simulink model "Problem5"  (R2016a)
settings: Solver=VariableStepAuto  StartTime=0.0  StopTime=.2  RelTol=1e-3
values from neighbouring files (symbols this model uses):
  f_sw = 10e3    (= 10000)    [EE487_HW4.m]
  If_desired = Vbus/((P/2)*Maf*wr)    (= 1.9098593171)    [EE487_HW4.m]
  K_i_a = 100    [EE487_HW4.m]
  K_i_f = 100    [EE487_HW4.m]
  K_p_a = 100    [EE487_HW4.m]
  K_p_f = 100    [EE487_HW4.m]
  La = 1e-3    (= 0.001)    [EE487_HW4.m]
  Lf = 200e-3    (= 0.2)    [EE487_HW4.m]
  Maf = 40e-3    (= 0.04)    [EE487_HW4.m]
  P = 4    [EE487_HW4.m]
  Ra = 1e-3    (= 0.001)    [EE487_HW4.m]
  Rf = 20    [EE487_HW4.m]
  T_step = 5    [EE487_HW4.m]
  Vbus = 48    [EE487_HW4.m]
  wr = (2*pi*rpm)/60    (= 314.159265359)    [EE487_HW4.m]
libraries: dspsigops x3
settings Model: Creator=Seth Barger  LastModifiedBy=Seth Barger

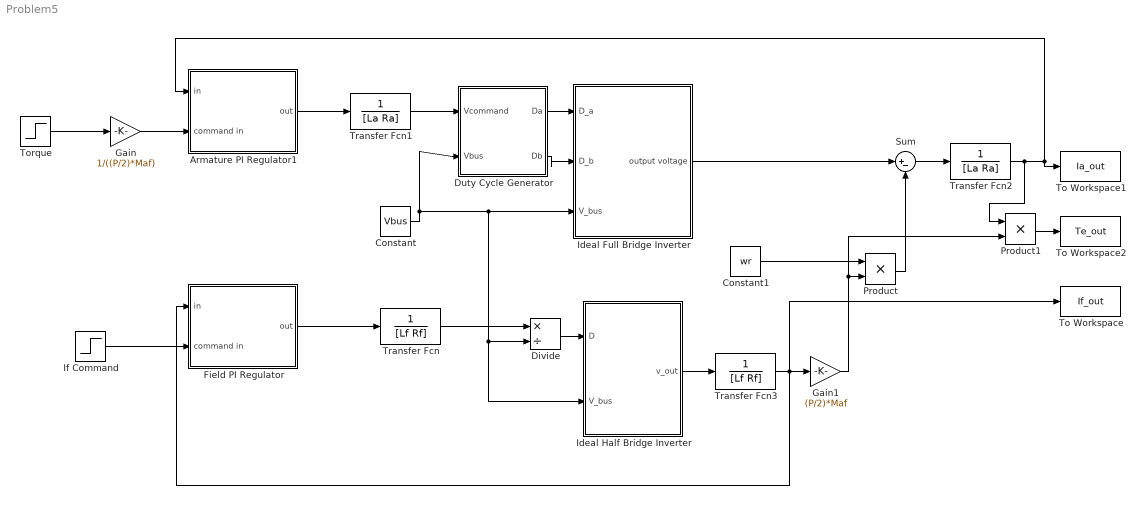
== system Problem5 ==
  Armature PI Regulator1 : Subsystem
  Constant : Constant  Value=Vbus
  Constant1 : Constant  Value=wr
  Divide : Product  Inputs=*/
  "Duty Cycle Generator " : Subsystem
  Field PI Regulator : Subsystem
  Gain : Gain  Gain=1/((P/2)*Maf)
  Gain1 : Gain  Gain=(P/2)*Maf
  "Ideal Half Bridge Inverter " : Subsystem
  "Ideal Full Bridge Inverter " : Subsystem
  If Command : Step  Time=.002  After=If_desired  SampleTime=0
  Product : Product
  Product1 : Product
  Sum : Sum  Inputs=|+-
  To Workspace : ToWorkspace  VariableName=If_out  SampleTime=-1
  To Workspace1 : ToWorkspace  VariableName=Ia_out  SampleTime=-1
  To Workspace2 : ToWorkspace  VariableName=Te_out  SampleTime=-1
  Torque : Step  Time=.002  After=T_step  SampleTime=0
  Transfer Fcn : TransferFcn  Denominator=[Lf Rf]
  Transfer Fcn1 : TransferFcn  Denominator=[La Ra]
  Transfer Fcn2 : TransferFcn  Denominator=[La Ra]
  Transfer Fcn3 : TransferFcn  Denominator=[Lf Rf]
  wires:
  "Duty Cycle Generator "/1(Da) -> "Ideal Full Bridge Inverter "/1(D_a)
  "Duty Cycle Generator "/2(Db) -> "Ideal Full Bridge Inverter "/2(D_b)
  Divide/1 -> "Ideal Half Bridge Inverter "/1(D)
  Constant/1 -> "Ideal Half Bridge Inverter "/2(V_bus), Divide/2, "Ideal Full Bridge Inverter "/3(V_bus), "Duty Cycle Generator "/2(Vbus)
  Field PI Regulator/1(out) -> Transfer Fcn/1
  Transfer Fcn/1 -> Divide/1
  Transfer Fcn1/1 -> "Duty Cycle Generator "/1(Vcommand)
  "Ideal Half Bridge Inverter "/1(v_out) -> Transfer Fcn3/1
  Transfer Fcn3/1 -> To Workspace/1, Gain1/1, Field PI Regulator/1(in)
  Transfer Fcn2/1 -> Product1/1, Armature PI Regulator1/1(in), To Workspace1/1
  If Command/1 -> Field PI Regulator/2(command in)
  Gain/1 -> Armature PI Regulator1/2(command in)
  Torque/1 -> Gain/1
  Armature PI Regulator1/1(out) -> Transfer Fcn1/1
  "Ideal Full Bridge Inverter "/1(output voltage) -> Sum/1
  Constant1/1 -> Product/1
  Product/1 -> Sum/2
  Sum/1 -> Transfer Fcn2/1
  Product1/1 -> To Workspace2/1
  Gain1/1 -> Product1/2, Product/2

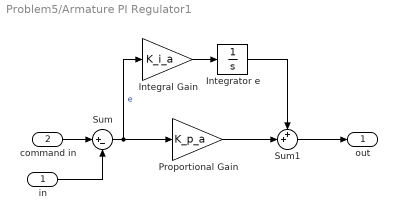
== system Problem5/Armature PI Regulator1 ==
  in : Inport
  command in : Inport  Port=2
  Integral Gain : Gain  Gain=K_i_a  SaturateOnIntegerOverflow=on  OutDataTypeStr=Inherit: Same as input  ParamDataTypeStr=Inherit: Same as input
  Integrator e : Integrator
  Proportional Gain : Gain  Gain=K_p_a  SaturateOnIntegerOverflow=on  OutDataTypeStr=Inherit: Same as input  ParamDataTypeStr=Inherit: Same as input
  Sum : Sum  Inputs=|+-  SaturateOnIntegerOverflow=on
  Sum1 : Sum  Inputs=++|  SaturateOnIntegerOverflow=on
  out : Outport
  wires:
  Sum/1 -> Integral Gain/1, Proportional Gain/1  "e"
  command in/1 -> Sum/1
  in/1 -> Sum/2
  Proportional Gain/1 -> Sum1/2
  Sum1/1 -> out/1
  Integral Gain/1 -> Integrator e/1
  Integrator e/1 -> Sum1/1

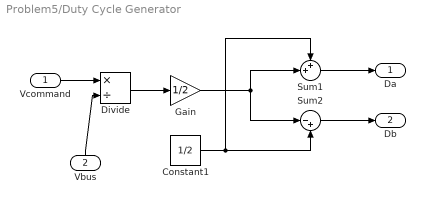
== system Problem5/Duty Cycle Generator  ==
  Vcommand : Inport
  Vbus : Inport  Port=2
  Constant1 : Constant  Value=1/2
  Divide : Product  Inputs=*/
  Gain : Gain  Gain=1/2
  Sum1 : Sum  Inputs=++|
  Sum2 : Sum  Inputs=|-+
  Da : Outport
  Db : Outport  Port=2
  wires:
  Divide/1 -> Gain/1
  Vcommand/1 -> Divide/1
  Gain/1 -> Sum2/1, Sum1/2
  Constant1/1 -> Sum1/1, Sum2/2
  Sum1/1 -> Da/1
  Sum2/1 -> Db/1
  Vbus/1 -> Divide/2

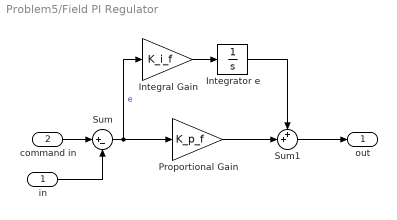
== system Problem5/Field PI Regulator ==
  in : Inport
  command in : Inport  Port=2
  Integral Gain : Gain  Gain=K_i_f  SaturateOnIntegerOverflow=on  OutDataTypeStr=Inherit: Same as input  ParamDataTypeStr=Inherit: Same as input
  Integrator e : Integrator
  Proportional Gain : Gain  Gain=K_p_f  SaturateOnIntegerOverflow=on  OutDataTypeStr=Inherit: Same as input  ParamDataTypeStr=Inherit: Same as input
  Sum : Sum  Inputs=|+-  SaturateOnIntegerOverflow=on
  Sum1 : Sum  Inputs=++|  SaturateOnIntegerOverflow=on
  out : Outport
  wires:
  Sum/1 -> Integral Gain/1, Proportional Gain/1  "e"
  command in/1 -> Sum/1
  in/1 -> Sum/2
  Proportional Gain/1 -> Sum1/2
  Sum1/1 -> out/1
  Integral Gain/1 -> Integrator e/1
  Integrator e/1 -> Sum1/1

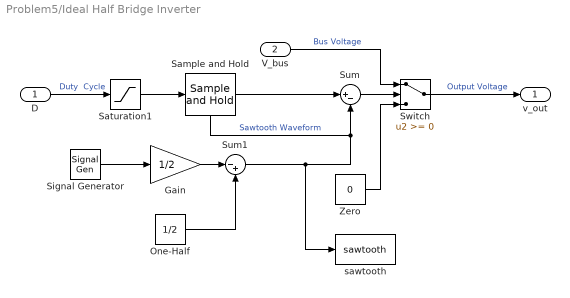
== system Problem5/Ideal Half Bridge Inverter  ==
  D : Inport
  V_bus : Inport  Port=2
  Gain : Gain  Gain=1/2  SaturateOnIntegerOverflow=on  OutDataTypeStr=Inherit: Same as input  ParamDataTypeStr=Inherit: Same as input
  One-Half : Constant  Value=1/2
  Sample and Hold : dspsigops/Sample and Hold  trig=Falling edge  initCond=0  latchinput=off
  Saturation1 : Saturate  UpperLimit=1  LowerLimit=0
  Signal Generator : SignalGenerator  WaveForm=sawtooth  Frequency=10e3
  Sum : Sum  Inputs=|+-  SaturateOnIntegerOverflow=on
  Sum1 : Sum  Inputs=|-+  SaturateOnIntegerOverflow=on
  Switch : Switch  SaturateOnIntegerOverflow=on
  Zero : Constant  Value=0
  sawtooth : ToWorkspace  VariableName=sawtooth  SampleTime=-1
  v_out : Outport
  wires:
  Sum1/1 -> Sample and Hold/Trigger, Sum/2, sawtooth/1  "Sawtooth Waveform"
  Sum/1 -> Switch/2
  Zero/1 -> Switch/3
  V_bus/1 -> Switch/1  "Bus Voltage"
  Switch/1 -> v_out/1  "Output Voltage"
  Signal Generator/1 -> Gain/1
  Gain/1 -> Sum1/1
  One-Half/1 -> Sum1/2
  D/1 -> Saturation1/1  "Duty  Cycle"
  Sample and Hold/1 -> Sum/1
  Saturation1/1 -> Sample and Hold/1

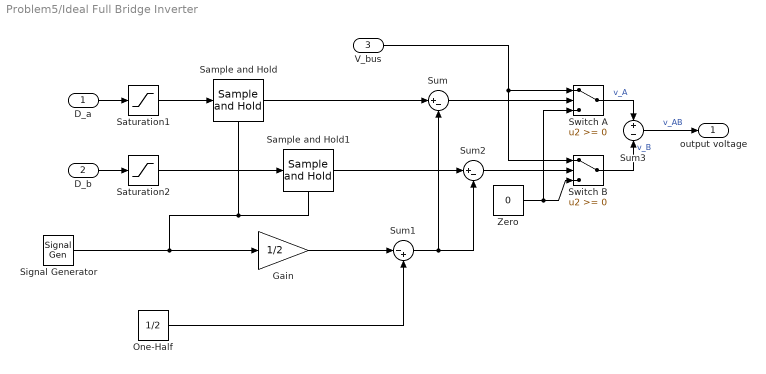
== system Problem5/Ideal Full Bridge Inverter  ==
  D_a : Inport
  D_b : Inport  Port=2
  V_bus : Inport  Port=3
  Gain : Gain  Gain=1/2  SaturateOnIntegerOverflow=on  OutDataTypeStr=Inherit: Same as input  ParamDataTypeStr=Inherit: Same as input
  One-Half : Constant  Value=1/2
  Sample and Hold : dspsigops/Sample and Hold  trig=Falling edge  initCond=0  latchinput=off
  Sample and Hold1 : dspsigops/Sample and Hold  trig=Falling edge  initCond=0  latchinput=off
  Saturation1 : Saturate  UpperLimit=1  LowerLimit=0
  Saturation2 : Saturate  UpperLimit=1  LowerLimit=0
  Signal Generator : SignalGenerator  WaveForm=sawtooth  Frequency=f_sw
  Sum : Sum  Inputs=|+-  SaturateOnIntegerOverflow=on
  Sum1 : Sum  Inputs=|-+  SaturateOnIntegerOverflow=on
  Sum2 : Sum  Inputs=|+-  SaturateOnIntegerOverflow=on
  Sum3 : Sum  Inputs=+-  SaturateOnIntegerOverflow=on
  Switch A : Switch  SaturateOnIntegerOverflow=on
  Switch B : Switch  SaturateOnIntegerOverflow=on
  Zero : Constant  Value=0
  output voltage : Outport
  wires:
  Sum/1 -> Switch A/2
  Zero/1 -> Switch A/3, Switch B/3
  Signal Generator/1 -> Sample and Hold/Trigger, Sample and Hold1/Trigger, Gain/1
  Gain/1 -> Sum1/1
  One-Half/1 -> Sum1/2
  Sum2/1 -> Switch B/2
  Switch A/1 -> Sum3/1  "v_A"
  Switch B/1 -> Sum3/2  "v_B"
  Sum3/1 -> output voltage/1  "v_AB"
  Sum1/1 -> Sum2/2, Sum/2
  V_bus/1 -> Switch A/1, Switch B/1
  D_a/1 -> Saturation1/1
  Sample and Hold/1 -> Sum/1
  D_b/1 -> Saturation2/1
  Sample and Hold1/1 -> Sum2/1
  Saturation1/1 -> Sample and Hold/1
  Saturation2/1 -> Sample and Hold1/1
